simulink model "simulation"  (R2022b)
settings: Solver=VariableStepAuto  StartTime=0.0  StopTime=10.0  RelTol=1e-3
values from neighbouring files (symbols this model uses):
  a = -1/taux    (= -62.5)    [variable.m]
  b = context.isCodeGenTarget('rtw')    [DCMotor2Set.m]    (also in variable.m = 3311.25)
  kI = K(2)    [variable.m]
  kX = K(1)    [variable.m]
  L = transpose(Ltrans)    [variable.m]
undefined symbols (not defined in the file or in its folder): A0, B0, C0, sigbuilder_block
settings Model: Creator=lgoudal  LastModifiedBy=lgoudal

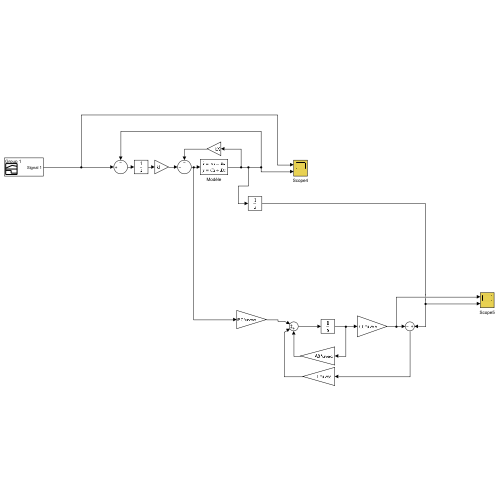
[thumbnail: Simulink's stored preview of the top-level diagram]
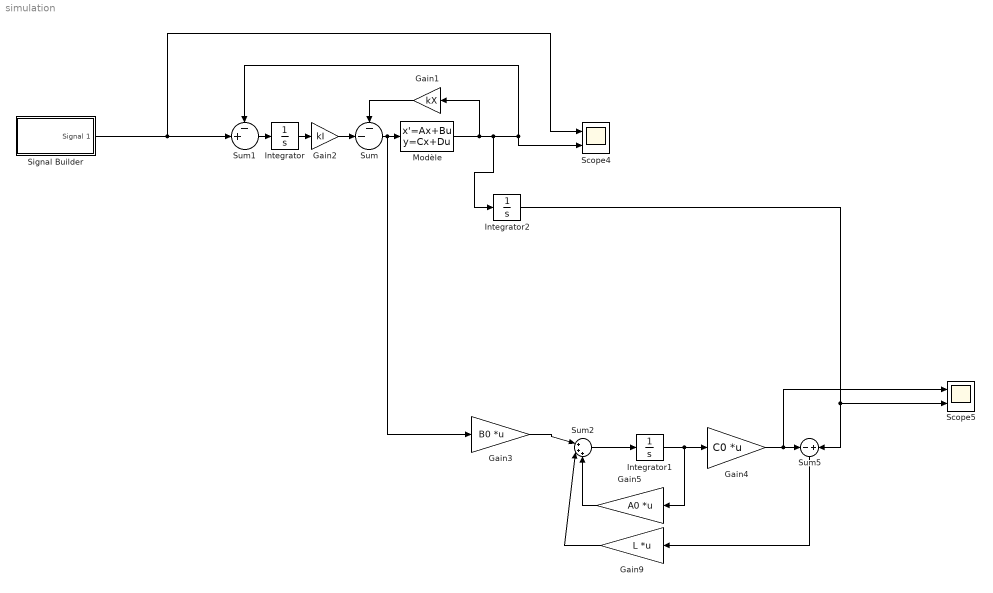
== system simulation ==
  Gain1 : Gain  Gain=kX
  Gain2 : Gain  Gain=kI
  Gain3 : Gain  Gain=B0  Multiplication=Matrix(K*u) (u vector)
  Gain4 : Gain  Gain=C0  Multiplication=Matrix(K*u) (u vector)
  Gain5 : Gain  Gain=A0  Multiplication=Matrix(K*u) (u vector)
  Gain9 : Gain  Gain=L  Multiplication=Matrix(K*u) (u vector)
  Integrator : Integrator
  Integrator1 : Integrator
  Integrator2 : Integrator
  Modèle : StateSpace  A=a-10  B=b-250  D=0  InitialCondition=0
  Scope4 : Scope  NumInputPorts=2
  Scope5 : Scope  NumInputPorts=2
  Signal Builder : Subsystem  Tag=STV Subsys  LoadFcn=sigbuilder_block('load');  StartFcn=sigbuilder_block('start');  StopFcn=sigbuilder_block('stop');  ClipboardFcn=sigbuilder_block('clipboard');  mask(Sigbuilder block){tuvar=[0:10]}
      mask help: Simulink:masks:SigbuilderBlock_MD
      mask init:
      | if ~strcmp(get_param(bdroot(gcbh),'SimulationStatus'),'stopped') tuvar = sigbuilder_block('maskInit'); end
      settings: CopyFcn=sigbuilder_block('copy');  DeleteFcn=sigbuilder_block('delete');  ModelCloseFcn=sigbuilder_block('modelClose');  PreSaveFcn=sigbuilder_block('preSave');  PauseFcn=sigbuilder_block('pause');  ContinueFcn=sigbuilder_block('continue');  NameChangeFcn=sigbuilder_block('namechange');  OpenFcn=sigbuilder_block('open',[382.125 217.125 550.5 400.5 ]);  CloseFcn=sigbuilder_block('close');
      mask Display: plot(0, 0, 100, 100,[2, 2, 32, 32, 2], [68, 8, 8, 68, 68],[32, 2], [38, 38], [32, 19, 2],[53, 60, 44], [32, 17, 17, 2],[16, 16, 31, 31]);txt = getActiveGroup(gcbh);text(2, 100, txt,'verticalAlignment', 'top');
  Sum : Sum  Inputs=--|
  Sum1 : Sum  Inputs=-+|
  Sum2 : Sum  Inputs=|+++
  Sum5 : Sum  Inputs=-|+
  wires:
  Integrator/1 -> Gain2/1
  Modèle/1 -> Integrator2/1, Scope4/2, Sum1/1, Gain1/1
  Gain2/1 -> Sum/2
  Gain1/1 -> Sum/1
  Sum1/1 -> Integrator/1
  Signal Builder/1(Signal 1) -> Scope4/1, Sum1/2
  Sum/1 -> Gain3/1, Modèle/1
  Gain9/1 -> Sum2/2
  Integrator1/1 -> Gain5/1, Gain4/1
  Gain4/1 -> Scope5/1, Sum5/1
  Sum2/1 -> Integrator1/1
  Gain3/1 -> Sum2/1
  Integrator2/1 -> Sum5/2, Scope5/2
  Gain5/1 -> Sum2/3
  Sum5/1 -> Gain9/1

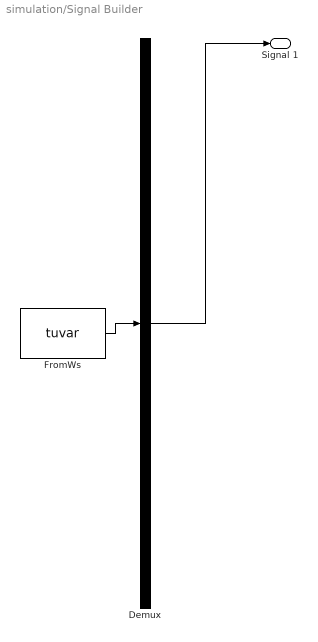
== system simulation/Signal Builder ==
  Demux : Demux  Tag=STV Demux  Outputs=1
      settings: DisplayOption=none
  FromWs : FromWorkspace  Tag=STV FromWs  VariableName=tuvar
      SigBuilderData=|
      | common.afterFinalStr = 'Extrapolate'
      | common.sampleTime = 0
      | dataSet.timeRange = [0 10]
      | dataSet.name = 'Group 1'
      | sbobj.Groups.Name = 'Group 1'
      | sbobj.Groups.Signals.Name = 'Signal 1'
      | sbobj.Groups.Signals.XData = [0 1 1 1.5 1.5 4 4 5 5 7 7 8 8 9 9 9.5 9.5 10]
      | sbobj.Groups.Signals.YData = [0 0 7 7 0 0 4 4 0 0 -4 -4 0 0 -7 -7 0 0]
  Signal 1 : Outport  Tag=STV Outport  VectorParamsAs1DForOutWhenUnconnected=off
  wires:
  Demux/1 -> Signal 1/1
  FromWs/1 -> Demux/1
